simulink model "Grid_connected_three_phase_inverter"  (R2023a)
settings: Solver=FixedStepDiscrete  StartTime=0.0  StopTime=0.1  FixedStep=SampleTime  RelTol=1e-3  AbsTol=1e-3
InitFcn:
  | SampleTime = 1e-6;
  | 
  | Pn = 20e3;
  | En = 400;
  | Udc = 800;
  | f0 = 50;
  | 
  | L1 = 2e-3;
  | Cdc = 2000e-6;
  | Rdc = 32;
  | fsw = 10e3;
  | Tc = 1/fsw;
  | 
  | Curr_Kp = 4.43612657703582;
  | Curr_Ki = 2045.91501898325;
  | 
  | Volt_Kp = 2.1671;
  | Volt_Ki = 164.2462;
libraries: ee_lib x13, nesl_utility x12, eeTransforms x6, fl_lib x4, slpidlib x3, eeSinusoidalMeasurementV2 x2, eeGeneralControl x2, eePwmGeneratorTwoLevel x2
settings Model: Creator=asus  LastModifiedBy=asus
settings SolverCC: AutoScaleAbsTol=off  AlgebraicLoopSolver=TrustRegion  MaxZcPerStep=1
settings DebuggingCC: UnconnectedInputMsg=warning  UnconnectedOutputMsg=warning  UnconnectedLineMsg=warning  SymbolicDimsDataTypeCodeGenerationDiagnostic=none
settings ModelReferenceCC: EnableRefExpFcnMdlSchedulingChecks=on
settings SFSimCC: CustomCodeUndefinedFunction=UseInterfaceOnly
settings RTWCC: DLArmComputeVersion=19.05
settings SimscapeCC: SimscapeLogType=all  SimscapeLogSimulationStatistics=on  SimscapeLogDataHistory=10000

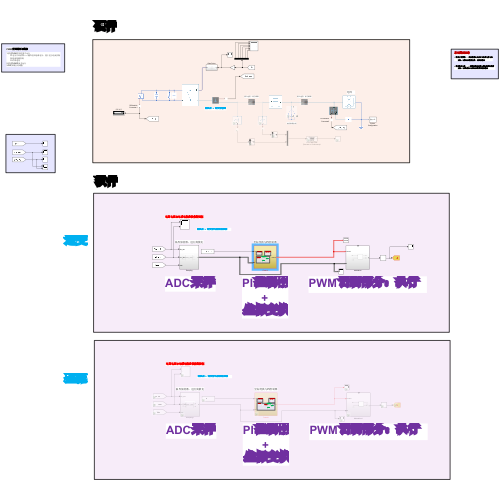
[thumbnail: Simulink's stored preview of the top-level diagram]
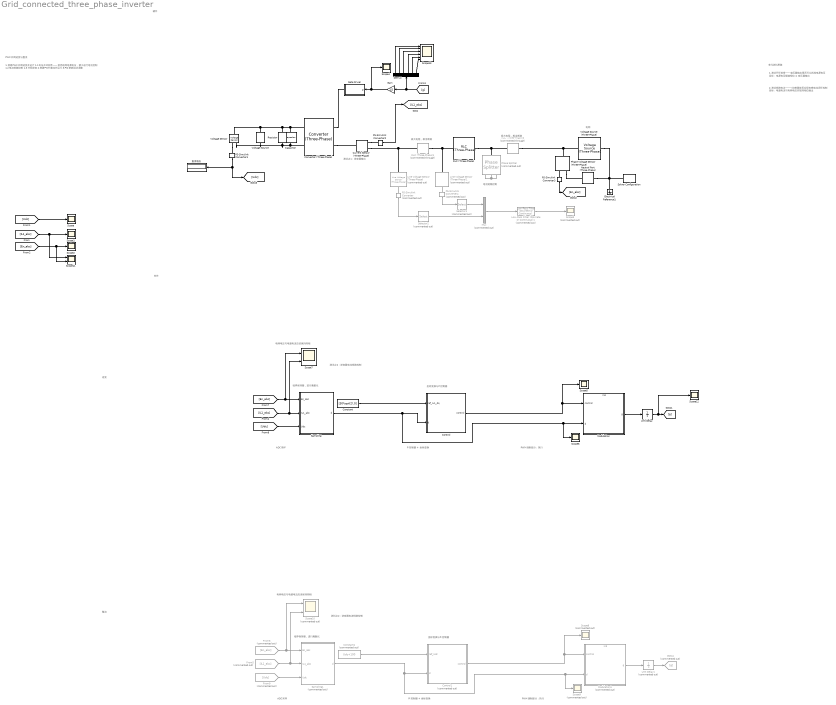
== system Grid_connected_three_phase_inverter ==
  note: 逆变
  note: 软件
  note: 2.测试短路电流------PI控制器能否实现电感电流闭环控制
      | 目标：电感电流与电网电压实现同相位输出
  note: ADC采样
  note: 电网电压与电感电流应该保持同相
  note: 电流短路控制
  note: 极大电阻，相当断路
  note: 测试点1：逆变器输出
  note: 1.测试开环前馈------变压器输出是否可以抵挡电源电压
      | 目标：电源电压幅值相位 = 变压器输出
  note: 单元测试思路
  note: 临界保持器，进行离散化
  note: 电网
  note: 1.搭建PWM并网逆变并运行
      | 1.1电压开环前馈------抵挡电网电源电压，便于进行电流控制
      | 1.2电流短路控制
      | 1.3并网逆变
      | 2.搭建PWM整流并运行
      | 3.PID参数自动调整
  note: PWM并网逆变与整流
  note: 坐标变换与PI控制器
  note: 极大电阻，相当断路
  note: PI控制器
      | +
      | 坐标变换
  note: PWM调制部分：执行
  note: 测试点2：逆变器电流短路控制
  note: 硬件
  note: ADC采样
  note: 电网电压与电感电流应该保持同相
  note: 临界保持器，进行离散化
  note: 坐标变换与PI控制器
  note: PI控制器
      | +
      | 坐标变换
  note: PWM调制部分：执行
  note: 测试点2：逆变器电流短路控制
  note: 整流
  Capacitor : fl_lib/Electrical/Electrical Elements/Capacitor  c=Cdc F  r=1e-6 Ohm  g=0 1/Ohm  i_specify=off  i_priority=None  i=0 A  i_nominal_specify=off  i_nominal_unit=A  i_nominal_value=1  v_specify=on  v_priority=None  v=Udc V  v_nominal_specify=off  v_nominal_unit=V  v_nominal_value=1  vc_specify=on  vc_priority=High  vc=Udc V  vc_nominal_specify=off  vc_nominal_unit=V  vc_nominal_value=1
  Constant : Constant  Value=[30*sqrt(2),0]
  Constant1 : Constant  Commented=on  Value=Udc+100
  Control : Subsystem
  Control1 : Subsystem  Commented=on
  Converter (Three-Phase) : ee_lib/Semiconductors & Converters/Converters/Converter (Three-Phase)  port_option=ee.enum.threePhasePort.composite  device_type=ee.enum.converters.switchingdevice.mosfet  K=0  Vf=0.8 V  Ron=0.001 Ohm  Rds=0.001 Ohm  Goff=1e-6 1/Ohm  Vgt=1 V  Vgt_off=-1 V  Ih=1 A  Vth=6 V  diode_param=ee.enum.converters.protectiondiode.nodynamics  diode_Vf=0.8 V  diode_Ron=0.001 Ohm  diode_Goff=1e-5 1/Ohm  diode_C=50 nF  diode_iRM=-235 A  diode_iF=300 A  diode_idot=-50 A/us  diode_trr_param=ee.enum.converters.diodetrr.trr_factor  diode_trr_factor=3  diode_trr=15 us  diode_Qrr=1500 s*uA  snubber_type=ee.enum.converters.snubber.exclude  Cs=1e-7 F  Rs=0.1 Ohm
  Current Sensor (Three-Phase) : ee_lib/Sensors & Transducers/Current Sensor (Three-Phase)
  Demux : Demux  Outputs=6
  Electrical Reference1 : fl_lib/Electrical/Electrical Elements/Electrical Reference
  From5 : From  Commented=on  GotoTag=IL1_abc
  From6 : From  Commented=on  GotoTag=En_abc
  From9 : From  Commented=on  GotoTag=Udc
  Gain : Gain  Gain=15
  Gate Drvier : Subsystem
  Goto4 : Goto  Commented=on  GotoTag=g
  Line Voltage Sensor (Three-Phase) : ee_lib/Sensors & Transducers/Line Voltage Sensor (Three-Phase)  Commented=on
  Line Voltage Sensor (Three-Phase)1 : ee_lib/Sensors & Transducers/Line Voltage Sensor (Three-Phase)  Commented=on
  Low-Pass Filter (Discrete or Continuous)1 : eeGeneralControl/Low-Pass Filter (Discrete or Continuous)  Commented=on  K=1  T=1/(500*2*pi)  B=inf  A=-inf  init_option=Inherited from block input  x0=0  Ts=-1
  Modulation : Subsystem
      settings: PortSchema="{\"entries\":[{\"content\":{\"sides\":[{\"content\":{\"connectorIds\":[\"In1\",\"In2\"]},\"type\":\"ConnectorPlacement.EquallySpacedRectSide\",\"uuid\":\"6f2b4e45-07a4-4b9a-b264-e657ed3e3d49\"},{\"content\":{\"connectorIds\":[\"Out1\"],\"side\":\"RIGHT\"},\"type\":\"ConnectorPlacement.EquallySpacedRectSide\",\"uuid\":\"fc619c4c-e947-4a72-af3b-717aea721804\"},{\"content\":{\"connectorIds\":[\"In3\"],\"side\":\"TOP\"},\"type\":\"ConnectorPlacement.EquallySpacedRectSide\",\"uuid\":\"14f31373-6e47-42c6-b65b-1061da0f8a55\"}]},\"type\":\"ConnectorPlacement.EquallySpacedConnector\",\"uuid\":\"2be9814a-ca60-4095-87d8-3ef7ff015fd2\"}],\"packageUris\":[\"http://schema.mathworks.com/mf0/Connector/R2020b\"],\"version\":\"1.0\"}"
  Modulation1 : Subsystem  Commented=on
      settings: PortSchema="{\"entries\":[{\"content\":{\"sides\":[{\"content\":{\"connectorIds\":[\"In1\",\"In2\"]},\"type\":\"ConnectorPlacement.EquallySpacedRectSide\",\"uuid\":\"6f2b4e45-07a4-4b9a-b264-e657ed3e3d49\"},{\"content\":{\"connectorIds\":[\"Out1\"],\"side\":\"RIGHT\"},\"type\":\"ConnectorPlacement.EquallySpacedRectSide\",\"uuid\":\"fc619c4c-e947-4a72-af3b-717aea721804\"},{\"content\":{\"connectorIds\":[\"In3\"],\"side\":\"TOP\"},\"type\":\"ConnectorPlacement.EquallySpacedRectSide\",\"uuid\":\"14f31373-6e47-42c6-b65b-1061da0f8a55\"}]},\"type\":\"ConnectorPlacement.EquallySpacedConnector\",\"uuid\":\"2be9814a-ca60-4095-87d8-3ef7ff015fd2\"}],\"packageUris\":[\"http://schema.mathworks.com/mf0/Connector/R2020b\"],\"version\":\"1.0\"}"
  Mux : Mux  Commented=on  Inputs=2
  Neutral Port (Three-Phase) : ee_lib/Connectors & References/Neutral Port (Three-Phase)  G_parasitic=1e-12 1/Ohm
      settings: InternalSimscapePortConfiguration="{\"Bottom\":[],\"Left\":[{\"id\":\"N\",\"label\":\"~\",\"type\":\"foundation.electrical.three_phase\"}],\"Right\":[{\"id\":\"n\",\"label\":\"n\",\"type\":\"foundation.electrical.electrical\"}],\"Top\":[]}"
  PS-Simulink Converter : nesl_utility/PS-Simulink Converter  Commented=on  PhysicalDomain=network_engine_domain  SubClassName=ps_output  LeftPortType=input  RightPortType=output  PseudoPeriodic=off  Frequencies=[]  VectorFormat=inherit  Unit=inherit  AffineConversion=off
  PS-Simulink Converter1 : nesl_utility/PS-Simulink Converter  PhysicalDomain=network_engine_domain  SubClassName=ps_output  LeftPortType=input  RightPortType=output  PseudoPeriodic=off  Frequencies=[]  VectorFormat=1-D array  Unit=inherit  AffineConversion=off
  PS-Simulink Converter2 : nesl_utility/PS-Simulink Converter  PhysicalDomain=network_engine_domain  SubClassName=ps_output  LeftPortType=input  RightPortType=output  PseudoPeriodic=off  Frequencies=[]  VectorFormat=1-D array  Unit=inherit  AffineConversion=off
  PS-Simulink Converter3 : nesl_utility/PS-Simulink Converter  PhysicalDomain=network_engine_domain  SubClassName=ps_output  LeftPortType=input  RightPortType=output  PseudoPeriodic=off  Frequencies=[]  VectorFormat=1-D array  Unit=inherit  AffineConversion=off
  PS-Simulink Converter4 : nesl_utility/PS-Simulink Converter  Commented=on  PhysicalDomain=network_engine_domain  SubClassName=ps_output  LeftPortType=input  RightPortType=output  PseudoPeriodic=off  Frequencies=[]  VectorFormat=inherit  Unit=inherit  AffineConversion=off
  Phase Splitter : ee_lib/Connectors & References/Phase Splitter  Commented=on
  Phase Voltage Sensor (Three-Phase) : ee_lib/Sensors & Transducers/Phase Voltage Sensor (Three-Phase)
  RLC (Three-Phase) : ee_lib/Passive/RLC Assemblies/RLC (Three-Phase)  component_structure=ee.enum.rlc.structure.L  R=1 Ohm  L=L1 H  C=1e-6 F  R_parasitic=0 Ohm  G_parasitic=0 1/Ohm  IL_specify=off  IL_priority=High  IL=[0, 0, 0] A  IL_nominal_specify=off  IL_nominal_unit=A  IL_nominal_value=1  VC_specify=off  VC_priority=High  VC=[0, 0, 0] V  VC_nominal_specify=off  VC_nominal_unit=V  VC_nominal_value=1
      settings: InternalSimscapePortConfiguration="{\"Bottom\":[],\"Left\":[{\"id\":\"N1\",\"label\":\"~1\",\"type\":\"foundation.electrical.three_phase\"}],\"Right\":[{\"id\":\"N2\",\"label\":\"~2\",\"type\":\"foundation.electrical.three_phase\"}],\"Top\":[]}"
  RLC (Three-Phase)1 : ee_lib/Passive/RLC Assemblies/RLC (Three-Phase)  Commented=through  component_structure=ee.enum.rlc.structure.R  R=100 MOhm  L=L1 H  C=1e-6 F  R_parasitic=0 Ohm  G_parasitic=0 1/Ohm  IL_specify=off  IL_priority=High  IL=[0, 0, 0] A  IL_nominal_specify=off  IL_nominal_unit=A  IL_nominal_value=1  VC_specify=off  VC_priority=High  VC=[0, 0, 0] V  VC_nominal_specify=off  VC_nominal_unit=V  VC_nominal_value=1
      settings: InternalSimscapePortConfiguration="{\"Bottom\":[],\"Left\":[{\"id\":\"N1\",\"label\":\"~1\",\"type\":\"foundation.electrical.three_phase\"}],\"Right\":[{\"id\":\"N2\",\"label\":\"~2\",\"type\":\"foundation.electrical.three_phase\"}],\"Top\":[]}"
  RLC (Three-Phase)2 : ee_lib/Passive/RLC Assemblies/RLC (Three-Phase)  Commented=through  component_structure=ee.enum.rlc.structure.R  R=100 MOhm  L=L1 H  C=1e-6 F  R_parasitic=0 Ohm  G_parasitic=0 1/Ohm  IL_specify=off  IL_priority=High  IL=[0, 0, 0] A  IL_nominal_specify=off  IL_nominal_unit=A  IL_nominal_value=1  VC_specify=off  VC_priority=High  VC=[0, 0, 0] V  VC_nominal_specify=off  VC_nominal_unit=V  VC_nominal_value=1
      settings: InternalSimscapePortConfiguration="{\"Bottom\":[],\"Left\":[{\"id\":\"N1\",\"label\":\"~1\",\"type\":\"foundation.electrical.three_phase\"}],\"Right\":[{\"id\":\"N2\",\"label\":\"~2\",\"type\":\"foundation.electrical.three_phase\"}],\"Top\":[]}"
  Resistor : fl_lib/Electrical/Electrical Elements/Resistor  R=Rdc*2 Ohm  i_specify=off  i_priority=None  i=0 A  i_nominal_specify=off  i_nominal_unit=A  i_nominal_value=1  v_specify=off  v_priority=None  v=0 V  v_nominal_specify=off  v_nominal_unit=V  v_nominal_value=1
  Sampling : Subsystem
  Sampling1 : Subsystem  Commented=on
  Scope{,1..2,4..6,12} (7 alike) : Scope
  Scope10 : Scope  Commented=on  NumInputPorts=2
  Scope11 : Scope  NumInputPorts=2
  Scope13 : Scope  NumInputPorts=6
  Scope3 : Scope  Commented=on
  Scope7 : Scope  NumInputPorts=2
  Scope8 : Scope  Commented=on
  Scope9 : Scope  Commented=on
  Selector1 : Selector  Commented=on  InputPortWidth=3  IndexOptions=Index vector (dialog)  Indices=[1]  OutputSizes=1
  Selector2 : Selector  Commented=on  InputPortWidth=3  IndexOptions=Index vector (dialog)  Indices=[1]  OutputSizes=1
  Solver Configuration : nesl_utility/Solver Configuration  PhysicalDomain=network_engine_domain  SubClassName=solver  LeftPortType=input  RightPortType=generic  Tones=[]  Harmonics=[]  SimulateNoise=off  Profile=off  UseLocalSampling=off  EnableSwitchedLinearOptims=on  FrequencyDomain=off  UseCCode=off  RelTol=0.001  AbsTol=1e-06  MinStep=1e-09  ToWorkspace=off  RevertToSquareIcSolve=off  NumHomotopyIterations=100  PhasorMode=off  PhasorModeNumHarmonics=1  ConsistencySolver=NEWTON_XTOL_AFTER_FTOL  IndexReductionMethod=DerivativeReplacement  DoDC=off  ResidualTolerance=1e-09  ConsistencyTolSource=GLOBAL  ConsistencyAbsTol=0.001  ConsistencyRelTol=0.001  ConsistencyTolFactor=0.001  UseLocalSolver=on  LocalSolverChoice=NE_BACKWARD_EULER_ADVANCER  ResolveIndetEquations=on  FunctionEvalNumThread=1  LocalSolverSampleTime=SampleTime  DoFixedCost=off  MaxNonlinIter=4  MaxModeIter=2  ComputeImpulses=off  ImpulseIterations=2  LinearAlgebra=auto  LinearAlgebraNumThread=0  EquationFormulation=NE_TIME_EF  DelaysMemoryBudget=1024  AutomaticFiltering=on  FilteringTimeConstant=0.001  PartitionStorageMethod=AS_NEEDED  PartitionMemoryBudget=1024  PartitionMethod=ROBUST
  Unit Delay : UnitDelay  SampleTime=-1  HasFrameUpgradeWarning=on
  Unit Delay1 : UnitDelay  Commented=on  SampleTime=-1  HasFrameUpgradeWarning=on
  Voltage Source (Three-Phase) : ee_lib/Sources/Voltage Source (Three-Phase)  vline_rms=En V  shift=0 deg  freq=f0 Hz  impedance_option=0  SShortCircuit=1e6 A*V  XR=15  R=0.01 Ohm  L=3.97e-4 H  harmonic_option=0  harmonic_orders=[5, 7, 11, 13]  harmonic_ratios=[.1, .1, .1, .1]  G_parasitic=0 1/Ohm  I_specify=off  I_priority=None  I=[0, 0, 0] A  I_nominal_specify=off  I_nominal_unit=A  I_nominal_value=1
  Voltage Sensor : fl_lib/Electrical/Electrical Sensors/Voltage Sensor
  Voltage Source : ee_lib/Sources/Voltage Source  dc_voltage=Udc V  ac_voltage=0 V  ac_shift=0 rad  ac_frequency=60 Hz  noise_mode=ee.enum.sources.noise.Disabled  PSD=0 V^2/Hz  sample_time=1e-3 s  repeatability=ee.enum.sources.repeatability.NotRepeatable  user_seed=0  auto_seed=3890346746  i_specify=off  i_priority=None  i=0 A  i_nominal_specify=off  i_nominal_unit=A  i_nominal_value=1  v_specify=off  v_priority=None  v=0 V  v_nominal_specify=off  v_nominal_unit=V  v_nominal_value=1
  直流电压 : Display
  wires:
  PS-Simulink Converter1/1 -> [Udc], 直流电压/1
  PS-Simulink Converter2/1 -> [IL1_abc]
  PS-Simulink Converter3/1 -> [En_abc]
  [Udc] -> Scope/1
  [IL1_abc] -> Scope11/1, Scope1/1
  [En_abc] -> Scope11/2, Scope2/1
  [g] -> Gain/1, Demux/1
  [En_abc] -> Scope7/1, Sampling/1(En_abc)
  [IL1_abc] -> Scope7/2, Sampling/2(IL1_abc)
  [Udc] -> Sampling/3(Udc)
  Sampling/1(d) -> Scope6/1, Modulation/2(d), Control/2(d)
  Constant/1 -> Control/1(ref_IL1_dq)
  Modulation/1(g) -> Unit Delay/1
  Unit Delay/1 -> Scope12/1, [g]
  Control/1(control) -> Modulation/1(control), Scope5/1
  PS-Simulink Converter4/1 -> Selector1/1
  PS-Simulink Converter/1 -> Selector2/1
  Mux/1 -> Low-Pass Filter (Discrete or Continuous)1/1
  Gain/1 -> Gate Drvier/1(g), Scope4/1
  Selector1/1 -> Mux/1
  Selector2/1 -> Mux/2
  Low-Pass Filter (Discrete or Continuous)1/1 -> Scope3/1
  Control1/1(control) -> Scope8/1, Modulation1/1(control)
  Unit Delay1/1 -> Goto4/1
  Modulation1/1(g) -> Unit Delay1/1
  Constant1/1 -> Control1/1(ref_Udc)
  Sampling1/1(d) -> Control1/2(d), Modulation1/2(d), Scope9/1
  From9/1 -> Sampling1/3(Udc)
  From5/1 -> Sampling1/2(IL1_abc), Scope10/2
  From6/1 -> Sampling1/1(En_abc), Scope10/1
  Demux/1 -> Scope13/1
  Demux/2 -> Scope13/2
  Demux/3 -> Scope13/3
  Demux/4 -> Scope13/4
  Demux/5 -> Scope13/5
  Demux/6 -> Scope13/6
  connections:
  Converter (Three-Phase)/RConn1 -- Voltage Sensor/LConn1 -- Voltage Source/LConn1 -- Resistor/LConn1 -- Capacitor/LConn1
  Phase Voltage Sensor (Three-Phase)/LConn1 -- RLC (Three-Phase)2/RConn1 -- Voltage Source (Three-Phase)/RConn1
  Converter (Three-Phase)/LConn2 -- Current Sensor (Three-Phase)/LConn1
  Voltage Source (Three-Phase)/LConn1 -- Solver Configuration/RConn1 -- Neutral Port (Three-Phase)/RConn1 -- Electrical Reference1/LConn1
  Phase Voltage Sensor (Three-Phase)/RConn2 -- Neutral Port (Three-Phase)/LConn1
  Converter (Three-Phase)/LConn1 -- Gate Drvier/RConn1
  Voltage Sensor/RConn1 -- PS-Simulink Converter1/LConn1
  Current Sensor (Three-Phase)/RConn1 -- PS-Simulink Converter2/LConn1
  PS-Simulink Converter3/LConn1 -- Phase Voltage Sensor (Three-Phase)/RConn1
  RLC (Three-Phase)1/RConn1 -- RLC (Three-Phase)/LConn1 -- Line Voltage Sensor (Three-Phase)1/LConn1
  Current Sensor (Three-Phase)/RConn2 -- Line Voltage Sensor (Three-Phase)/LConn1 -- RLC (Three-Phase)1/LConn1
  PS-Simulink Converter/LConn1 -- Line Voltage Sensor (Three-Phase)/RConn1
  PS-Simulink Converter4/LConn1 -- Line Voltage Sensor (Three-Phase)1/RConn1
  RLC (Three-Phase)/RConn1 -- Phase Splitter/LConn1 -- RLC (Three-Phase)2/LConn1
  Phase Splitter/RConn3 -- Phase Splitter/RConn2 -- Phase Splitter/RConn1
  Converter (Three-Phase)/RConn2 -- Voltage Source/RConn1 -- Voltage Sensor/RConn2 -- Resistor/RConn1 -- Capacitor/RConn1

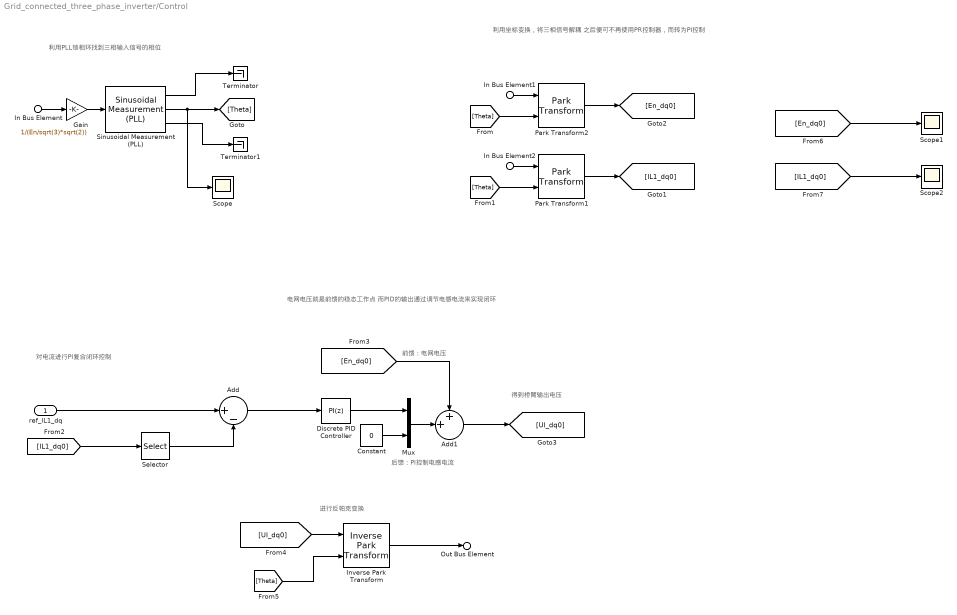
== system Grid_connected_three_phase_inverter/Control ==
  note: 后馈：PI控制电感电流
  note: 前馈：电网电压
  note: 对电流进行PI复合闭环控制
  note: 利用PLL锁相环找到三相输入信号的相位
  note: 利用坐标变换，将三相信号解耦
      | 之后便可不再使用PR控制器，而转为PI控制
  note: 电网电压就是前馈的稳态工作点
      | 而PID的输出通过调节电感电流来实现闭环
  note: 得到桥臂输出电压
  note: 进行反帕克变换
  ref_IL1_dq : Inport
  In Bus Element : Inport  Port=2  PortName=d  Element=En_abc
  In Bus Element1 : Inport  Port=2  PortName=d  Element=En_abc
  In Bus Element2 : Inport  Port=2  PortName=d  Element=IL1_abc
  Add : Sum  Inputs=|+-
  Add1 : Sum  Inputs=++|
  Constant : Constant  Value=0
  Discrete PID Controller : slpidlib/PID Controller  Controller=PI  Form=Parallel  TimeDomain=Discrete-time  UseExternalTs=off  SampleTime=-1  IntegratorMethod=Forward Euler  FilterMethod=Forward Euler  ControllerParametersSource=internal  P=Curr_Kp  I=Curr_Ki  UseKiTs=off  D=0  N=100  UseFilter=on  TunerSelectOption=Transfer Function Based (PID Tuner App)  InitialConditionSource=internal  InitialConditionForIntegrator=0  InitialConditionForFilter=0  DifferentiatorICPrevScaledInput=0  ExternalReset=none  TrackingMode=off  Kt=1  LimitOutput=on  SatLimitsSource=internal  UpperSaturationLimit=60  LowerSaturationLimit=-60  LinearizeAsGain=off  AntiWindupMode=clamping  Kb=1  LimitIntegrator=off  UpperIntegratorSaturationLimit=inf  LowerIntegratorSaturationLimit=-inf  POutMin=[]  POutMax=[]  IOutMin=[]  IOutMax=[]  DOutMin=[]  DOutMax=[]  NOutMin=[]  NOutMax=[]  SumOutMin=[]  SumOutMax=[]  SaturationOutMin=[]  SaturationOutMax=[]  PParamMin=[]  PParamMax=[]  IParamMin=[]  IParamMax=[]  DParamMin=[]  DParamMax=[]  NParamMin=[]  NParamMax=[]  KbParamMin=[]  KbParamMax=[]  KtParamMin=[]  KtParamMax=[]  KbOutMin=[]  KbOutMax=[]  KtOutMin=[]  KtOutMax=[]  IntegratorOutMin=[]  IntegratorOutMax=[]  FilterOutMin=[]  FilterOutMax=[]  SumI1OutMin=[]  SumI1OutMax=[]  SumI2OutMin=[]  SumI2OutMax=[]  SumI3OutMin=[]  SumI3OutMax=[]  SumI4OutMin=[]  SumI4OutMax=[]  SumDOutMin=[]  SumDOutMax=[]  DifferentiatorOutMin=[]  DifferentiatorOutMax=[]  FilterDiffOutCoefMin=[]  FilterDiffOutCoefMax=[]  ReciprocalOutMin=[]  ReciprocalOutMax=[]  SumDenOutMin=[]  SumDenOutMax=[]  SumNumOutMin=[]  SumNumOutMax=[]  DivideOutMin=[]  DivideOutMax=[]  UdiffTsProdOutMin=[]  UdiffTsProdOutMax=[]  NTsProdOutMin=[]  NTsProdOutMax=[]  UintegralTsProdOutMin=[]  UintegralTsProdOutMax=[]  UngainTsProdOutMin=[]  UngainTsProdOutMax=[]  ClampingZeroOutDataTypeStr=Inherit: Inherit via back propagation  ClampingZeroOutMin=[]  ClampingZeroOutMax=[]  FilterDenConstantOutDataTypeStr=Inherit: Inherit via back propagation  FilterDenConstantOutMin=[]  FilterDenConstantOutMax=[]  PCopyOutDataTypeStr=Inherit: Inherit via back propagation  PCopyOutMin=[]  PCopyOutMax=[]  NCopyOutDataTypeStr=Inherit: Inherit via back propagation  NCopyOutMin=[]  NCopyOutMax=[]  IntegratorContinuousStateAttributes=''  IntegratorStateMustResolveToSignalObject=off  IntegratorRTWStateStorageClass=Auto  FilterContinuousStateAttributes=''  FilterStateMustResolveToSignalObject=off  FilterRTWStateStorageClass=Auto  ParallelPVariant=InternalParameters  IdealPVariant=Disabled  IVariant=InternalParameters  DVariant=Disabled  IntegratorVariant=Discrete  SatVariant=Enabled  AWVariant=DiscClampingParallel  PCopyVariant=Disabled  TRVariant=Disabled  FdbkBlocksVariant=Forward  IdealPFdbkVariant=Disabled  SatFdbkVariant=Disabled  DerivativeFilterVariant=Disabled  NVariant=Disabled  NCopyVariant=Disabled_SignalSpec  FilterICVariant=Disabled  IntegratorICVariant=InternalICs  ExternalResetVariant=Disabled  TRSumVariant=Passthrough  SumFdbkVariant=Disabled  SumVariant=Sum_PI  TsampFilterVariant=InternalTs  TsampNgainVariant=Passthrough  TsampIntegralVariant=Disabled_SignalSpec  ExternalSaturationOutDataTypeStr=Inherit: Same as second input
      settings: LibrarySourceBlock=simulink/Discrete/Discrete PID Controller
  Gain : Gain  Gain=1/(En/sqrt(3)*sqrt(2))
  Inverse Park Transform : eeTransforms/Inverse Park Transform  AxisAlignment=Q-axis  PowerInvariant=off
      settings: LibrarySourceBlock=|
      | ee_sl_lib/Mathematical
      | Transforms/Inverse
      | Park Transform
  Mux : Mux  Inputs=2
  Park Transform1 : eeTransforms/Park Transform  AxisAlignment=Q-axis  PowerInvariant=off
      settings: LibrarySourceBlock=|
      | ee_sl_lib/Mathematical
      | Transforms/Park Transform
  Park Transform2 : eeTransforms/Park Transform  AxisAlignment=Q-axis  PowerInvariant=off
      settings: LibrarySourceBlock=|
      | ee_sl_lib/Mathematical
      | Transforms/Park Transform
  Scope : Scope
  Scope1 : Scope
  Scope2 : Scope
  Selector : Selector  InputPortWidth=3  IndexOptions=Index vector (dialog)  Indices=[1 2]  OutputSizes=1
  Sinusoidal Measurement (PLL) : eeSinusoidalMeasurementV2/Sinusoidal Measurement (PLL)  Ki_PD=1000  Kp_LF=400  Ki_LF=20000  F0=50  Theta0=0  Mag0=1  Ts=-1
      settings: LibrarySourceBlock=|
      | ee_sl_lib/Measurements/Sinusoidal Measurement
      | (PLL)
  Terminator : Terminator
  Terminator1 : Terminator
  Out Bus Element : Outport  PortName=control  Element=UI_abc
  wires:
  In Bus Element/1 -> Gain/1
  Gain/1 -> Sinusoidal Measurement (PLL)/1
  Sinusoidal Measurement (PLL)/1 -> Terminator/1
  Sinusoidal Measurement (PLL)/3 -> Terminator1/1
  Sinusoidal Measurement (PLL)/2 -> Scope/1, [Theta]
  In Bus Element1/1 -> Park Transform2/1
  [Theta] -> Park Transform2/2
  In Bus Element2/1 -> Park Transform1/1
  [Theta] -> Park Transform1/2
  Park Transform1/1 -> [IL1_dq0]
  Park Transform2/1 -> [En_dq0]
  ref_IL1_dq/1 -> Add/1
  [IL1_dq0] -> Selector/1
  Selector/1 -> Add/2
  Add/1 -> Discrete PID Controller/1
  Discrete PID Controller/1 -> Mux/1
  Constant/1 -> Mux/2
  Add1/1 -> [UI_dq0]
  [UI_dq0] -> Inverse Park Transform/1
  [Theta] -> Inverse Park Transform/2
  Inverse Park Transform/1 -> Out Bus Element/1
  Mux/1 -> Add1/2
  [En_dq0] -> Add1/1
  [En_dq0] -> Scope1/1
  [IL1_dq0] -> Scope2/1

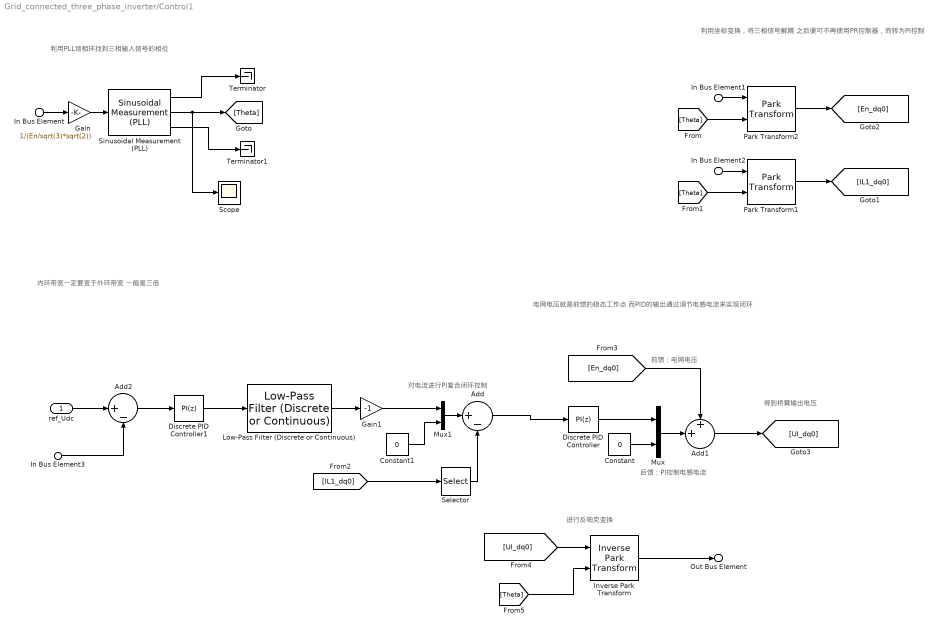
== system Grid_connected_three_phase_inverter/Control1 ==
  note: 内环带宽一定要宽于外环带宽
      | 一般是三倍
  note: 进行反帕克变换
  note: 得到桥臂输出电压
  note: 电网电压就是前馈的稳态工作点
      | 而PID的输出通过调节电感电流来实现闭环
  note: 利用坐标变换，将三相信号解耦
      | 之后便可不再使用PR控制器，而转为PI控制
  note: 利用PLL锁相环找到三相输入信号的相位
  note: 对电流进行PI复合闭环控制
  note: 前馈：电网电压
  note: 后馈：PI控制电感电流
  ref_Udc : Inport
  In Bus Element : Inport  Port=2  PortName=d  Element=En_abc
  In Bus Element1 : Inport  Port=2  PortName=d  Element=En_abc
  In Bus Element2 : Inport  Port=2  PortName=d  Element=IL1_abc
  In Bus Element3 : Inport  Port=2  PortName=d  Element=Udc
  Add : Sum  Inputs=|+-
  Add1 : Sum  Inputs=++|
  Add2 : Sum  Inputs=|+-
  Constant : Constant  Value=0
  Constant1 : Constant  Value=0
  Discrete PID Controller : slpidlib/PID Controller  Controller=PI  Form=Parallel  TimeDomain=Discrete-time  UseExternalTs=off  SampleTime=-1  IntegratorMethod=Forward Euler  FilterMethod=Forward Euler  ControllerParametersSource=internal  P=Curr_Kp  I=Curr_Ki  UseKiTs=off  D=0  N=100  UseFilter=on  TunerSelectOption=Transfer Function Based (PID Tuner App)  InitialConditionSource=internal  InitialConditionForIntegrator=0  InitialConditionForFilter=0  DifferentiatorICPrevScaledInput=0  ExternalReset=none  TrackingMode=off  Kt=1  LimitOutput=on  SatLimitsSource=internal  UpperSaturationLimit=60  LowerSaturationLimit=-60  LinearizeAsGain=off  AntiWindupMode=clamping  Kb=1  LimitIntegrator=off  UpperIntegratorSaturationLimit=inf  LowerIntegratorSaturationLimit=-inf  POutMin=[]  POutMax=[]  IOutMin=[]  IOutMax=[]  DOutMin=[]  DOutMax=[]  NOutMin=[]  NOutMax=[]  SumOutMin=[]  SumOutMax=[]  SaturationOutMin=[]  SaturationOutMax=[]  PParamMin=[]  PParamMax=[]  IParamMin=[]  IParamMax=[]  DParamMin=[]  DParamMax=[]  NParamMin=[]  NParamMax=[]  KbParamMin=[]  KbParamMax=[]  KtParamMin=[]  KtParamMax=[]  KbOutMin=[]  KbOutMax=[]  KtOutMin=[]  KtOutMax=[]  IntegratorOutMin=[]  IntegratorOutMax=[]  FilterOutMin=[]  FilterOutMax=[]  SumI1OutMin=[]  SumI1OutMax=[]  SumI2OutMin=[]  SumI2OutMax=[]  SumI3OutMin=[]  SumI3OutMax=[]  SumI4OutMin=[]  SumI4OutMax=[]  SumDOutMin=[]  SumDOutMax=[]  DifferentiatorOutMin=[]  DifferentiatorOutMax=[]  FilterDiffOutCoefMin=[]  FilterDiffOutCoefMax=[]  ReciprocalOutMin=[]  ReciprocalOutMax=[]  SumDenOutMin=[]  SumDenOutMax=[]  SumNumOutMin=[]  SumNumOutMax=[]  DivideOutMin=[]  DivideOutMax=[]  UdiffTsProdOutMin=[]  UdiffTsProdOutMax=[]  NTsProdOutMin=[]  NTsProdOutMax=[]  UintegralTsProdOutMin=[]  UintegralTsProdOutMax=[]  UngainTsProdOutMin=[]  UngainTsProdOutMax=[]  ClampingZeroOutDataTypeStr=Inherit: Inherit via back propagation  ClampingZeroOutMin=[]  ClampingZeroOutMax=[]  FilterDenConstantOutDataTypeStr=Inherit: Inherit via back propagation  FilterDenConstantOutMin=[]  FilterDenConstantOutMax=[]  PCopyOutDataTypeStr=Inherit: Inherit via back propagation  PCopyOutMin=[]  PCopyOutMax=[]  NCopyOutDataTypeStr=Inherit: Inherit via back propagation  NCopyOutMin=[]  NCopyOutMax=[]  IntegratorContinuousStateAttributes=''  IntegratorStateMustResolveToSignalObject=off  IntegratorRTWStateStorageClass=Auto  FilterContinuousStateAttributes=''  FilterStateMustResolveToSignalObject=off  FilterRTWStateStorageClass=Auto  ParallelPVariant=InternalParameters  IdealPVariant=Disabled  IVariant=InternalParameters  DVariant=Disabled  IntegratorVariant=Discrete  SatVariant=Enabled  AWVariant=DiscClampingParallel  PCopyVariant=Disabled  TRVariant=Disabled  FdbkBlocksVariant=Forward  IdealPFdbkVariant=Disabled  SatFdbkVariant=Disabled  DerivativeFilterVariant=Disabled  NVariant=Disabled  NCopyVariant=Disabled_SignalSpec  FilterICVariant=Disabled  IntegratorICVariant=InternalICs  ExternalResetVariant=Disabled  TRSumVariant=Passthrough  SumFdbkVariant=Disabled  SumVariant=Sum_PI  TsampFilterVariant=InternalTs  TsampNgainVariant=Passthrough  TsampIntegralVariant=Disabled_SignalSpec  ExternalSaturationOutDataTypeStr=Inherit: Same as second input
      settings: LibrarySourceBlock=simulink/Discrete/Discrete PID Controller
  Discrete PID Controller1 : slpidlib/PID Controller  Controller=PI  Form=Parallel  TimeDomain=Discrete-time  UseExternalTs=off  SampleTime=-1  IntegratorMethod=Forward Euler  FilterMethod=Forward Euler  ControllerParametersSource=internal  P=Volt_Kp  I=Volt_Ki  UseKiTs=off  D=0  N=100  UseFilter=on  TunerSelectOption=Frequency Response Based  InitialConditionSource=internal  InitialConditionForIntegrator=0  InitialConditionForFilter=0  DifferentiatorICPrevScaledInput=0  ExternalReset=none  TrackingMode=off  Kt=1  LimitOutput=on  SatLimitsSource=internal  UpperSaturationLimit=30*sqrt(2)  LowerSaturationLimit=-30*sqrt(2)  LinearizeAsGain=off  AntiWindupMode=clamping  Kb=1  LimitIntegrator=off  UpperIntegratorSaturationLimit=inf  LowerIntegratorSaturationLimit=-inf  POutMin=[]  POutMax=[]  IOutMin=[]  IOutMax=[]  DOutMin=[]  DOutMax=[]  NOutMin=[]  NOutMax=[]  SumOutMin=[]  SumOutMax=[]  SaturationOutMin=[]  SaturationOutMax=[]  PParamMin=[]  PParamMax=[]  IParamMin=[]  IParamMax=[]  DParamMin=[]  DParamMax=[]  NParamMin=[]  NParamMax=[]  KbParamMin=[]  KbParamMax=[]  KtParamMin=[]  KtParamMax=[]  KbOutMin=[]  KbOutMax=[]  KtOutMin=[]  KtOutMax=[]  IntegratorOutMin=[]  IntegratorOutMax=[]  FilterOutMin=[]  FilterOutMax=[]  SumI1OutMin=[]  SumI1OutMax=[]  SumI2OutMin=[]  SumI2OutMax=[]  SumI3OutMin=[]  SumI3OutMax=[]  SumI4OutMin=[]  SumI4OutMax=[]  SumDOutMin=[]  SumDOutMax=[]  DifferentiatorOutMin=[]  DifferentiatorOutMax=[]  FilterDiffOutCoefMin=[]  FilterDiffOutCoefMax=[]  ReciprocalOutMin=[]  ReciprocalOutMax=[]  SumDenOutMin=[]  SumDenOutMax=[]  SumNumOutMin=[]  SumNumOutMax=[]  DivideOutMin=[]  DivideOutMax=[]  UdiffTsProdOutMin=[]  UdiffTsProdOutMax=[]  NTsProdOutMin=[]  NTsProdOutMax=[]  UintegralTsProdOutMin=[]  UintegralTsProdOutMax=[]  UngainTsProdOutMin=[]  UngainTsProdOutMax=[]  ClampingZeroOutDataTypeStr=Inherit: Inherit via back propagation  ClampingZeroOutMin=[]  ClampingZeroOutMax=[]  FilterDenConstantOutDataTypeStr=Inherit: Inherit via back propagation  FilterDenConstantOutMin=[]  FilterDenConstantOutMax=[]  PCopyOutDataTypeStr=Inherit: Inherit via back propagation  PCopyOutMin=[]  PCopyOutMax=[]  NCopyOutDataTypeStr=Inherit: Inherit via back propagation  NCopyOutMin=[]  NCopyOutMax=[]  IntegratorContinuousStateAttributes=''  IntegratorStateMustResolveToSignalObject=off  IntegratorRTWStateStorageClass=Auto  FilterContinuousStateAttributes=''  FilterStateMustResolveToSignalObject=off  FilterRTWStateStorageClass=Auto  ParallelPVariant=InternalParameters  IdealPVariant=Disabled  IVariant=InternalParameters  DVariant=Disabled  IntegratorVariant=Discrete  SatVariant=Enabled  AWVariant=DiscClampingParallel  PCopyVariant=Disabled  TRVariant=Disabled  FdbkBlocksVariant=Forward  IdealPFdbkVariant=Disabled  SatFdbkVariant=Disabled  DerivativeFilterVariant=Disabled  NVariant=Disabled  NCopyVariant=Disabled_SignalSpec  FilterICVariant=Disabled  IntegratorICVariant=InternalICs  ExternalResetVariant=Disabled  TRSumVariant=Passthrough  SumFdbkVariant=Disabled  SumVariant=Sum_PI  TsampFilterVariant=InternalTs  TsampNgainVariant=Passthrough  TsampIntegralVariant=Disabled_SignalSpec  ExternalSaturationOutDataTypeStr=Inherit: Same as second input
      settings: LibrarySourceBlock=simulink/Discrete/Discrete PID Controller
  Gain : Gain  Gain=1/(En/sqrt(3)*sqrt(2))
  Gain1 : Gain  Gain=-1
  Inverse Park Transform : eeTransforms/Inverse Park Transform  AxisAlignment=Q-axis  PowerInvariant=off
      settings: LibrarySourceBlock=|
      | ee_sl_lib/Mathematical
      | Transforms/Inverse
      | Park Transform
  Low-Pass Filter (Discrete or Continuous) : eeGeneralControl/Low-Pass Filter (Discrete or Continuous)  K=1  T=1/(100*2*pi)  B=30*sqrt(2)  A=-30*sqrt(2)  init_option=Inherited from block input  x0=0  Ts=-1
  Mux : Mux  Inputs=2
  Mux1 : Mux  Inputs=2
  Park Transform1 : eeTransforms/Park Transform  AxisAlignment=Q-axis  PowerInvariant=off
      settings: LibrarySourceBlock=|
      | ee_sl_lib/Mathematical
      | Transforms/Park Transform
  Park Transform2 : eeTransforms/Park Transform  AxisAlignment=Q-axis  PowerInvariant=off
      settings: LibrarySourceBlock=|
      | ee_sl_lib/Mathematical
      | Transforms/Park Transform
  Scope : Scope
  Selector : Selector  InputPortWidth=3  IndexOptions=Index vector (dialog)  Indices=[1 2]  OutputSizes=1
  Sinusoidal Measurement (PLL) : eeSinusoidalMeasurementV2/Sinusoidal Measurement (PLL)  Ki_PD=1000  Kp_LF=400  Ki_LF=20000  F0=50  Theta0=0  Mag0=1  Ts=-1
      settings: LibrarySourceBlock=|
      | ee_sl_lib/Measurements/Sinusoidal Measurement
      | (PLL)
  Terminator : Terminator
  Terminator1 : Terminator
  Out Bus Element : Outport  PortName=control  Element=UI_abc
  wires:
  [En_dq0] -> Add1/1
  Mux/1 -> Add1/2
  Inverse Park Transform/1 -> Out Bus Element/1
  [Theta] -> Inverse Park Transform/2
  [UI_dq0] -> Inverse Park Transform/1
  Add1/1 -> [UI_dq0]
  Constant/1 -> Mux/2
  Discrete PID Controller/1 -> Mux/1
  Add/1 -> Discrete PID Controller/1
  Selector/1 -> Add/2
  [IL1_dq0] -> Selector/1
  Park Transform2/1 -> [En_dq0]
  Park Transform1/1 -> [IL1_dq0]
  [Theta] -> Park Transform1/2
  In Bus Element2/1 -> Park Transform1/1
  [Theta] -> Park Transform2/2
  In Bus Element1/1 -> Park Transform2/1
  Sinusoidal Measurement (PLL)/2 -> [Theta], Scope/1
  Sinusoidal Measurement (PLL)/3 -> Terminator1/1
  Sinusoidal Measurement (PLL)/1 -> Terminator/1
  Gain/1 -> Sinusoidal Measurement (PLL)/1
  In Bus Element/1 -> Gain/1
  ref_Udc/1 -> Add2/1
  In Bus Element3/1 -> Add2/2
  Low-Pass Filter (Discrete or Continuous)/1 -> Gain1/1
  Discrete PID Controller1/1 -> Low-Pass Filter (Discrete or Continuous)/1
  Add2/1 -> Discrete PID Controller1/1
  Mux1/1 -> Add/1
  Gain1/1 -> Mux1/1
  Constant1/1 -> Mux1/2

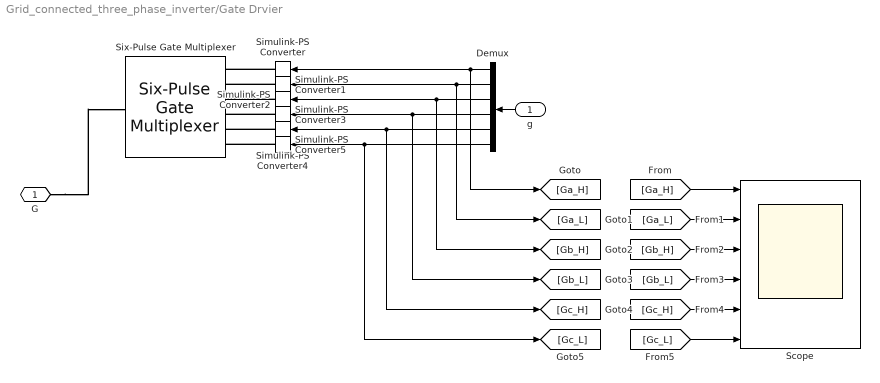
== system Grid_connected_three_phase_inverter/Gate Drvier ==
  g : Inport
  Demux : Demux  Outputs=6
  Scope : Scope  NumInputPorts=6
  Simulink-PS Converter{,1..5} (6 alike) : nesl_utility/Simulink-PS Converter  PhysicalDomain=network_engine_domain  SubClassName=ps_input  LeftPortType=input  RightPortType=output  PseudoPeriodic=off  Frequencies=[]  NoiseDistribution=none  NoiseParameters=[]  Unit=1  AffineConversion=off  FilteringAndDerivatives=provide  SimscapeFilterOrder=1  InputFilterTimeConstant=0.001  UdotUserProvided=0
  Six-Pulse Gate Multiplexer : ee_lib/Semiconductors & Converters/Converters/Six-Pulse Gate Multiplexer  port_option=ee.enum.controlport.ps
  G : PMIOPort  Side=Right
  wires:
  Demux/4 -> [Gb_L], Simulink-PS Converter3/1
  Demux/6 -> Simulink-PS Converter5/1, [Gc_L]
  Demux/2 -> Simulink-PS Converter1/1, [Ga_L]
  g/1 -> Demux/1
  Demux/1 -> Simulink-PS Converter/1, [Ga_H]
  Demux/3 -> [Gb_H], Simulink-PS Converter2/1
  Demux/5 -> Simulink-PS Converter4/1, [Gc_H]
  [Ga_H] -> Scope/1
  [Ga_L] -> Scope/2
  [Gb_H] -> Scope/3
  [Gb_L] -> Scope/4
  [Gc_H] -> Scope/5
  [Gc_L] -> Scope/6
  connections:
  G/RConn1 -- Six-Pulse Gate Multiplexer/RConn1
  Simulink-PS Converter/RConn1 -- Six-Pulse Gate Multiplexer/LConn1
  Simulink-PS Converter1/RConn1 -- Six-Pulse Gate Multiplexer/LConn2
  Simulink-PS Converter2/RConn1 -- Six-Pulse Gate Multiplexer/LConn3
  Simulink-PS Converter3/RConn1 -- Six-Pulse Gate Multiplexer/LConn4
  Simulink-PS Converter4/RConn1 -- Six-Pulse Gate Multiplexer/LConn5
  Simulink-PS Converter5/RConn1 -- Six-Pulse Gate Multiplexer/LConn6

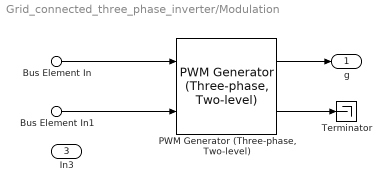
== system Grid_connected_three_phase_inverter/Modulation ==
  Bus Element In : Inport  PortName=control  Element=UI_abc
  Bus Element In1 : Inport  Port=2  PortName=d  Element=Udc
  In3 : Inport  Port=3
  "PWM Generator (Three-phase, Two-level)" : eePwmGeneratorTwoLevel/PWM Generator (Three-phase, Two-level)  PWMMode=Continuous PWM (CPWM)  CPWMMode=SPWM: sinusoidal PWM  DPWMMode=60 DPWM: 60 degree discontinuous PWM  fsw=fsw  Ts=SampleTime
      settings: SamplingMode=Asymmetric
      settings: LibrarySourceBlock=|
      | ee_sl_lib/Pulse Width
      | Modulation/PWM Generator
      | (Three-phase, Two-level)
  Terminator : Terminator
  g : Outport
  wires:
  Bus Element In/1 -> "PWM Generator (Three-phase, Two-level)"/1
  Bus Element In1/1 -> "PWM Generator (Three-phase, Two-level)"/2
  "PWM Generator (Three-phase, Two-level)"/2 -> Terminator/1
  "PWM Generator (Three-phase, Two-level)"/1 -> g/1

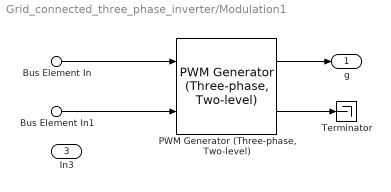
== system Grid_connected_three_phase_inverter/Modulation1 ==
  Bus Element In : Inport  PortName=control  Element=UI_abc
  Bus Element In1 : Inport  Port=2  PortName=d  Element=Udc
  In3 : Inport  Port=3
  "PWM Generator (Three-phase, Two-level)" : eePwmGeneratorTwoLevel/PWM Generator (Three-phase, Two-level)  PWMMode=Continuous PWM (CPWM)  CPWMMode=SPWM: sinusoidal PWM  DPWMMode=60 DPWM: 60 degree discontinuous PWM  fsw=fsw  Ts=SampleTime
      settings: SamplingMode=Asymmetric
      settings: LibrarySourceBlock=|
      | ee_sl_lib/Pulse Width
      | Modulation/PWM Generator
      | (Three-phase, Two-level)
  Terminator : Terminator
  g : Outport
  wires:
  "PWM Generator (Three-phase, Two-level)"/1 -> g/1
  "PWM Generator (Three-phase, Two-level)"/2 -> Terminator/1
  Bus Element In1/1 -> "PWM Generator (Three-phase, Two-level)"/2
  Bus Element In/1 -> "PWM Generator (Three-phase, Two-level)"/1

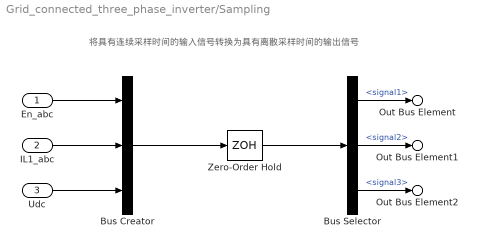
== system Grid_connected_three_phase_inverter/Sampling ==
  note: 将具有连续采样时间的输入信号转换为具有离散采样时间的输出信号
  En_abc : Inport
  IL1_abc : Inport  Port=2
  Udc : Inport  Port=3
  Bus Creator : BusCreator  Inputs=3
  Bus Selector : BusSelector  OutputSignals=signal1,signal2,signal3
  Zero-Order Hold : ZeroOrderHold  SampleTime=Tc
  Out Bus Element : Outport  PortName=d  Element=En_abc
  Out Bus Element1 : Outport  PortName=d  Element=IL1_abc
  Out Bus Element2 : Outport  PortName=d  Element=Udc
  wires:
  En_abc/1 -> Bus Creator/1
  IL1_abc/1 -> Bus Creator/2
  Udc/1 -> Bus Creator/3
  Bus Creator/1 -> Zero-Order Hold/1
  Zero-Order Hold/1 -> Bus Selector/1
  Bus Selector/1 -> Out Bus Element/1  "<signal1>"
  Bus Selector/2 -> Out Bus Element1/1  "<signal2>"
  Bus Selector/3 -> Out Bus Element2/1  "<signal3>"

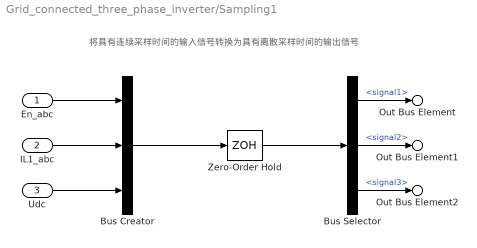
== system Grid_connected_three_phase_inverter/Sampling1 ==
  note: 将具有连续采样时间的输入信号转换为具有离散采样时间的输出信号
  En_abc : Inport
  IL1_abc : Inport  Port=2
  Udc : Inport  Port=3
  Bus Creator : BusCreator  Inputs=3
  Bus Selector : BusSelector  OutputSignals=signal1,signal2,signal3
  Zero-Order Hold : ZeroOrderHold  SampleTime=Tc
  Out Bus Element : Outport  PortName=d  Element=En_abc
  Out Bus Element1 : Outport  PortName=d  Element=IL1_abc
  Out Bus Element2 : Outport  PortName=d  Element=Udc
  wires:
  Bus Selector/3 -> Out Bus Element2/1  "<signal3>"
  Bus Selector/2 -> Out Bus Element1/1  "<signal2>"
  Bus Selector/1 -> Out Bus Element/1  "<signal1>"
  Zero-Order Hold/1 -> Bus Selector/1
  Bus Creator/1 -> Zero-Order Hold/1
  Udc/1 -> Bus Creator/3
  IL1_abc/1 -> Bus Creator/2
  En_abc/1 -> Bus Creator/1
